simulink model "Wind_Turbine"  (R2023a)
settings: Solver=VariableStepAuto  StartTime=0.0  StopTime=20000000  FixedStep=3600  RelTol=1e-2  AbsTol=1e-2  EnableMultiTasking=on
PreLoadFcn:
  | warning off Simulink:Commands:LoadMdlParameterizedLink
PostLoadFcn:
  | warning off Simulink:blocks:MatchingGotoNotFound
  | warning off Simulink:blocks:MatchingFromNotFound
  | warning('off','Simulink:SL_OutputNotConnected');
  | warning off Simulink:Engine:SaveWithParameterizedLinks_Warning
  | warning off Simulink:Engine:SaveWithDisabledLinks_Warning
  | warning('off','Simulink:fixpoint:fxpParameterPrecisionLoss');
  | warning off Simulink:blocks:DTConversionUncessary
  | warning off ne_sli:simulator:input:FilteredInputs
  | warning off MATLAB:nearlySingularMatrix
  | 
  | warning off xPCTarget:modeloptions:StackIncrease
  | warning off xPCTarget:sampleTime:sampleTimeInvariance
  | warning off Simulink:blocks:TDelayFixedBuffer
  | 
  | Setup_WT_Configurations
StartFcn:
  | tic
StopFcn:
  | Elapsed_Sim_Time = toc;
  | disp(['Elapsed time is ' num2str(Elapsed_Sim_Time)]);
undefined symbols (not defined in the file): Actuator_Lookup, radps2rpm, sigbuilder_block, WT_Params, X, Y, Z
libraries: sm_lib x6, fl_lib x5, Wind_Lib x4, nesl_utility x4, Yaw_System_Lib x4, Pitch_System_Lib x3, Pitch_Controller_Lib x3, spsGroundLib x2, spsThreePhaseVIMeasurementLib x2, Geartrain_Lib x2, spsThreePhaseSeriesRLCLoadLib x2, spsThreePhaseBreakerLib x2
(part 2 of 2)

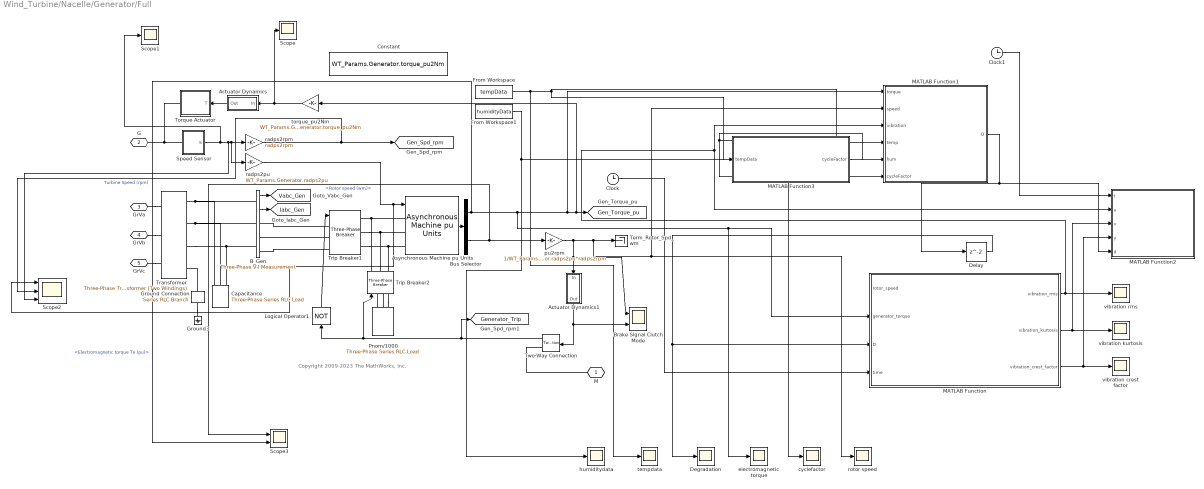
== system Wind_Turbine/Nacelle/Generator/Full ==
  note: Copyright 2009-2023 The MathWorks, Inc.
  Actuator Dynamics : Subsystem  mask(First-order lag supporting vector signals){b=WT_Params.Generator.generator_time_constant, x_initial=0}
      mask prompts: b "Filter time constant"; x_initial "Initial output"
      mask help: Models a lag of the form 1/(b*s+1) where s is the Laplace operator.
  Actuator Dynamics1 : Subsystem  mask(First-order lag supporting vector signals){b=WT_Params.Generator.generator_time_constant, x_initial=0}
      mask prompts: b "Filter time constant"; x_initial "Initial output"
      mask help: Models a lag of the form 1/(b*s+1) where s is the Laplace operator.
  Asynchronous Machine pu Units : spsAsynchronousMachinepuUnitsLib/Asynchronous Machine pu Units  RotorType=Squirrel-cage  PresetModel=No  MechanicalLoad=Speed w  ShowDetailedParameters=on  ReferenceFrame=Rotor  Units=pu  MeasurementBus=off  NominalParameters="[WT_Params.Generator.nominal_power  WT_Params.Generator.voltage WT_Params.Generator.frequency]"  VoltageRatio=1  Stator=[WT_Params.Generator.Stator.resistance WT_Params.Generator.Stator.inductance]  Rotor=[WT_Params.Generator.Rotor.resistance WT_Params.Generator.Rotor.inductance]  Cage1=[0.01909 0.0397]  Cage2=[0.01909 0.0397]  Lm=WT_Params.Generator.mutual_inductance  Mechanical=[0.09526 0.05479 3]  PolePairs=3  InitialConditions=[1 0 0 0 0 0 0 0]  SimulateSaturation=off  Saturation="[0.212,0.4201,0.8125,1.0979,1.4799,2.2457,3.2586,4.5763,6.4763 ;   0.5,0.7,0.9,1,1.1,1.2 ,1.3,1.4,1.5]"  LoadFlowParameters=1650000  TsPowergui=0  TsBlock=-1  IterativeModel=Forward Euler  IterativeDiscreteModel=Trapezoidal non iterative  Pmec=0
  B_Gen : spsThreePhaseVIMeasurementLib/Three-Phase V-I Measurement  VoltageMeasurement=phase-to-ground  SetLabelV=off  LabelV=Vabc  Vpu=on  VpuLL=off  CurrentMeasurement=yes  SetLabelI=off  LabelI=Iabc  Ipu=on  Pbase=WT_Params.Generator.nominal_power  Vbase=WT_Params.Generator.voltage  OutputType=Complex  PhasorSimulation=on  PSBequivalent=0
  Brake Signal Clutch Mode : Scope  NumInputPorts=2
  Bus Selector : BusSelector  OutputSignals=Mechanical.Electromagnetic torque Te (pu),Mechanical.Rotor speed (wm)
  Capacitance : spsThreePhaseSeriesRLCLoadLib/Three-Phase Series RLC Load  LConnTagsString=A|B|C  Configuration=Delta  NominalVoltage=WT_Params.Generator.voltage  Vabc=[1e3 1e3 1e3]  Vabcp=[1e3 1e3 1e3]  NominalFrequency=WT_Params.Generator.frequency  UnbalancedPower=off  ActivePower=0  InductivePower=0  CapacitivePower=200e3  Pabc=[10e3 9e3 11e3]  QLabc=[100 90 110]  QCabc=[100 90 110]  Pabcp=[10e3 9e3 11e3]  QLabcp=[100 90 110]  QCabcp=[100 90 110]  Measurements=None  LoadType=constant Z
  Clock : Clock
  Clock1 : Clock
  Constant : Constant  Value=WT_Params.Generator.torque_pu2Nm
  Degradation : Scope
  Delay : Delay  SampleTime=3600
  From Workspace : FromWorkspace  VariableName=tempData
  From Workspace1 : FromWorkspace  VariableName=humidityData
  Ground Connection : spsSeriesRLCBranchLib/Series RLC Branch  LConnTagsString=__new0  RConnTagsString=__new0  BranchType=R  Resistance=10  Inductance=1.0  SetiL0=off  InitialCurrent=0  Capacitance=1.0  Setx0=off  InitialVoltage=0  Measurements=None
  Ground3 : spsGroundLib/Ground  LConnTagsString=a
  Logical Operator1 : Logic  Operator=NOT  AllPortsSameDT=off  OutDataTypeStr=float('double')  SampleTime=0
  MATLAB Function : MATLAB Function  TreatAsAtomicUnit=on
  MATLAB Function1 : MATLAB Function  TreatAsAtomicUnit=on
  MATLAB Function2 : MATLAB Function  TreatAsAtomicUnit=on
  MATLAB Function3 : MATLAB Function  TreatAsAtomicUnit=on
  Pnom/1000 : spsThreePhaseSeriesRLCLoadLib/Three-Phase Series RLC Load  LConnTagsString=A|B|C  Configuration=Y (grounded)  NominalVoltage=WT_Params.Generator.voltage  Vabc=[1e3 1e3 1e3]  Vabcp=[1e3 1e3 1e3]  NominalFrequency=WT_Params.Generator.frequency  UnbalancedPower=off  ActivePower=WT_Params.Generator.nominal_power  InductivePower=0  CapacitivePower=0  Pabc=[10e3 9e3 11e3]  QLabc=[100 90 110]  QCabc=[100 90 110]  Pabcp=[10e3 9e3 11e3]  QLabcp=[100 90 110]  QCabcp=[100 90 110]  Measurements=None  LoadType=constant Z
  Scope : Scope
  Scope1 : Scope
  Scope2 : Scope  NumInputPorts=3
  Scope3 : Scope  NumInputPorts=2
  Speed Sensor : Subsystem
      mask Display:
      | plot([149.600878633536;150.016472378793;150.47508104106;150.972287968219;151.50330478576;152.063017511447;152.646035805762;153.246744883819;153.859359588817;154.477980106257;155.096648782383;155.709407499646;156.310355056631;156.893703999851;157.453836360095;157.985357756531;158.483149347555;158.942417128023;159.358738098149;159.728102859405;160.046954227227;160.312221488639;160.521349974904;160.672325664379;160.763694578642;160.794576785101;160.764674871227;160.674276808796;160.524253180566;160.316048796087;160.051668777399;159.733659248606;159.365082815313;158.949489070056;158.490880407788;157.993673480629;157.462656663088;156.908284800231], [156.971389291536;157.430657072004;157.84697804213;158.216342803387;158.535194171208;158.80046143262;159.009589918885;159.16056560836;159.251934522623;159.282816729083;159.252914815208;159.162516752777;159.012493124547;158.804288740068;158.53990872138;158.221899192587;157.853322759294;157.437729014037;156.979120351769;156.48191342461;155.950896607069;155.391183881382;154.808165587067;154.20745650901;153.594841804012;152.976221286573;152.357552610446;151.744793893183;151.143846336199;150.560497392978;150.000365032735;149.468843636298;148.971052045274;148.511784264806;148.095463294681;147.726098533424;147.407247165603;147.144199990631])
      | plot([152.057635404444;152.93604260309;153.834625296826;154.744729643097;155.657590839533;156.564417533794;157.45647648909;158.325176690034;159.162152078811;159.959342124889;160.709069452336;161.404113777147;162.037781442523;162.603969882449;163.097226392739;163.512800643557;163.846690427691;164.095680203997;164.257372064819;164.330208829146;164.313489039122;164.27939575172], [142.228020686971;141.979030910664;141.817339049842;141.744502285515;141.761222075539;141.867337399197;142.061826307913;142.342815767178;142.707599694895;143.152665022428;143.673725527376;144.265763112236;144.923076131425;145.639334301243;146.40763966397;147.220593018964;148.070365181011;148.948772379657;149.847355073393;150.757459419663;151.6703206161;152.055850472277])
      | plot([116.468514315784;116.438789536125;116.349901463023;116.202706137216;115.998621130155;115.739611892022;115.42817282337;115.067303252679;114.660478551187;114.211616663162;113.725040373958;113.205435679231;112.657806656235;112.087427271827;111.499790591278;110.900555877058;110.29549408704;109.690432297022;109.091197582803;108.503560902254;107.933181517846;107.38555249485;106.865947800123;106.379371510919;105.930509622894;105.523684921402;105.162815350711;104.851376282059;104.592367043926;104.388282036865;104.241086711057;104.152198637956;104.122473858297;104.152198637956;104.241086711057;104.388282036865;104.592367043926;104.851376282059;105.162815350711;105.523684921402;105.930509622894;106.379371510919;106.865947800123;107.38555249485;107.933181517846;108.503560902254;109.091197582803;109.690432297022;110.29549408704;110.900555877058;111.499790591278;112.087427271827;112.657806656235;113.205435679231;113.725040373958;114.211616663162;114.660478551187;115.067303252679;115.42817282337;115.739611892022;115.998621130155;116.202706137216;116.349901463023;116.438789536125;116.468514315784;116.468514315784], [111.618284136057;111.013222346039;110.413987631819;109.826350951271;109.255971566862;108.708342543866;108.188737849139;107.702161559936;107.253299671911;106.846474970419;106.485605399728;106.174166331075;105.915157092943;105.711072085881;105.563876760074;105.474988686973;105.445263907313;105.474988686973;105.563876760074;105.711072085881;105.915157092943;106.174166331075;106.485605399728;106.846474970419;107.253299671911;107.702161559936;108.188737849139;108.708342543866;109.255971566862;109.826350951271;110.413987631819;111.013222346039;111.618284136057;112.223345926075;112.822580640295;113.410217320843;113.980596705252;114.528225728247;115.047830422975;115.534406712178;115.983268600203;116.390093301695;116.750962872386;117.062401941038;117.321411179171;117.525496186232;117.67269151204;117.761579585141;117.7913043648;117.761579585141;117.67269151204;117.525496186232;117.321411179171;117.062401941038;116.750962872386;116.390093301695;115.983268600203;115.534406712178;115.047830422975;114.528225728247;113.980596705252;113.410217320843;112.822580640295;112.223345926075;111.618284136057;111.618284136057])
      | plot([239.23602886498;238.828071429858;237.608127977604;235.587947230552;232.78698463364;229.232214987837;224.957872668068;220.005121927465;214.421660463109;208.261260061133;201.583248745024;194.451939414329;186.936010476274;179.107844435155;171.042830809261;162.818640088593;154.514475725591;146.210311362589;137.986120641921;129.921107016027;122.092940974909;114.577012036853;107.445702706158;100.76769139005;94.607290988073;89.0238295237172;84.0710787831142;79.7967364633452;76.2419668175427;73.4410042206305;71.4208234735788;70.2008800213248;69.7929225862026;70.2008800213248;71.4208234735788;73.4410042206306;76.2419668175428;79.7967364633454;84.0710787831144;89.0238295237174;94.6072909880733;100.76769139005;107.445702706159;114.577012036853;122.092940974909;129.921107016027;137.986120641921;146.210311362589;154.514475725591;162.818640088593;171.042830809261;179.107844435155;186.936010476274;194.451939414329;201.583248745024;208.261260061133;214.421660463109;220.005121927465;224.957872668068;229.232214987837;232.78698463364;235.587947230552;237.608127977604;238.828071429858;239.23602886498;239.23602886498], [155.774275772274;147.47628550917;139.258209428443;131.199192095207;123.376846251889;115.866505365088;108.740498123116;102.067451871182;95.9116316925529;90.3323215006612;85.3832531026163;81.1120887325275;77.5599620381344;74.7610819412943;72.742403187363;71.5233667562631;71.1157126352191;71.5233667562631;72.742403187363;74.7610819412943;77.5599620381345;81.1120887325275;85.3832531026164;90.3323215006612;95.9116316925529;102.067451871182;108.740498123116;115.866505365089;123.376846251889;131.199192095207;139.258209428443;147.47628550917;155.774275772274;164.072266035377;172.290342116104;180.34935944934;188.171705292658;195.682046179459;202.808053421432;209.481099673365;215.636919851994;221.216230043886;226.165298441931;230.43646281202;233.988589506413;236.787469603253;238.806148357184;240.025184788284;240.432838909328;240.025184788284;238.806148357184;236.787469603253;233.988589506413;230.43646281202;226.165298441931;221.216230043886;215.636919851994;209.481099673365;202.808053421432;195.682046179459;188.171705292658;180.34935944934;172.290342116105;164.072266035378;155.774275772274;155.774275772274])
      | plot([252.715889364481;252.243022716633;250.828976737403;248.487369462568;245.240751850236;241.120390602797;236.165967051481;230.425195003451;223.953361231755;216.812793033479;209.072257983804;200.806301666664;192.094529760025;183.020841389688;173.672621134841;164.139897466795;154.514475725591;144.889053984387;135.356330316341;126.008110061494;116.934421691157;108.222649784518;99.9566934673787;92.2161584177032;85.075590219427;78.6037564477313;72.8629843997015;67.9085608483856;63.7881996009461;60.5415819886144;58.199974713779;56.7859287345493;56.3130620867014;56.7859287345493;58.1999747137791;60.5415819886146;63.7881996009463;67.9085608483858;72.8629843997018;78.6037564477315;85.0755902194273;92.2161584177035;99.9566934673791;108.222649784519;116.934421691157;126.008110061494;135.356330316341;144.889053984387;154.514475725591;164.139897466796;173.672621134841;183.020841389688;192.094529760025;200.806301666664;209.072257983803;216.812793033479;223.953361231755;230.425195003451;236.165967051481;241.120390602797;245.240751850236;248.487369462568;250.828976737403;252.243022716633;252.715889364481;252.715889364481], [154.514475725591;144.895228084285;135.36861905618;126.026395093992;116.958526921455;108.252343066071;99.9916888376535;92.2561188521535;85.1201308772245;78.6524483779929;72.9153586725213;67.9641130708855;63.8463947748555;60.6018596625959;58.2617543808809;56.8486154228053;56.3760520890355;56.8486154228053;58.2617543808809;60.6018596625959;63.8463947748555;67.9641130708856;72.9153586725213;78.652448377993;85.1201308772246;92.2561188521536;99.9916888376536;108.252343066072;116.958526921455;126.026395093992;135.36861905618;144.895228084285;154.514475725591;164.133723366898;173.660332395002;183.002556357191;192.070424529728;200.776608385111;209.037262613529;216.772832599029;223.908820573958;230.37650307319;236.113592778661;241.064838380297;245.182556676327;248.427091788587;250.767197070302;252.180336028377;252.652899362147;252.180336028377;250.767197070301;248.427091788587;245.182556676327;241.064838380297;236.113592778661;230.37650307319;223.908820573958;216.772832599029;209.037262613529;200.776608385111;192.070424529728;183.002556357191;173.660332395002;164.133723366898;154.514475725592;154.514475725591])
      | plot([154.514475725591;129.948374815285;179.017586633563;154.514475725591], [240.369848906994;203.583687543869;203.583687543869;240.369848906994])
      | plot([105.382273904979;149.60125554353], [115.271704271436;156.971085816622])
      | plot([144.688035361469;144.688035361469], [152.057865634561;203.583687543869])
      | plot([164.277926087379;164.277926087379], [152.057865634561;203.583687543869])
      | plot([159.112745895982;159.616665914655], [149.60125554353;149.60125554353])
      | plot([115.208714269102;159.364705905318], [107.901873998344;149.60125554353])
      | plot([0;311.800511553884;311.800511553884;0;0], [311.800511553884;311.800511553884;0;0;311.800511553884])
      | ;
      | color('red');
      | port_label('LConn', 1,'R')
      | port_label('output', 1,'W')
  Term_Rotor_Spd_wm : Terminator
  Torque Actuator : Subsystem
      mask Display:
      | plot([198.657636314574;187.5372000791;176.524559560751;165.725772507838;155.244837142898;145.182690602959;135.636236859729;126.697413481378;118.452306223496;110.980319976212;104.353414051689;98.6354091766174;93.8813728637222;90.1370890815176;87.4386173296598;85.811945366254;85.272738931537;85.8261908782356;87.4669711615554;90.1792781704262;93.9369909056548;98.7039205394262;104.434158933498;111.072520759669;118.555074964656;126.809760461083;135.75708011515;145.310866347487;155.379110974044;165.864851295207;176.667103899592;187.681837189509;192.988368326926], [283.691199740558;283.13774779386;281.49696751054;278.784660501669;275.026947766441;270.260018132669;264.529779738597;257.891417912426;250.40886370744;242.154178211013;233.206858556945;223.653072324609;213.584827698051;203.099087376889;192.296834772503;181.282101482586;170.160965409986;159.040529174513;148.027888656163;137.22910160325;126.748166238311;116.686019698372;107.139565955142;98.2007425767901;89.9556353189084;82.4836490716241;75.8567431471018;70.1387382720299;65.3847019591348;61.6404181769301;58.9419464250722;57.3152744616664;56.9214337615639])
      | plot([85.209725657478;1.11807254143059;1.11807254143059], [170.435198815539;170.435198815539;171.380048850551])
      | plot([283.691223012283;397.073227213696], [170.309218810871;170.309218810871])
      | plot([153.301918180659;255.34572196193], [170.309218810871;170.309218810871])
      | plot([198.654719861224;113.618216710165;198.654719861224], [85.2727156598121;170.309218810871;255.34572196193])
      | plot([198.654719861224;153.301918180659;198.654719861224], [215.662020491436;170.309218810871;124.956417130306])
      | plot([198.654719861224;283.691223012283;283.691223012283;187.316519441083;192.985619651154], [283.691223012283;283.691223012283;56.927214609459;56.927214609459;56.927214609459])
      | 
      | patch([395.419739652425;395.419739652425;5.6843418860808e-14;0;395.419739652425;394.947314634919;0.472425017505884;0.472425017505941;394.947314634919;394.947314634919;395.419739652425], [340.618437621742;5.6843418860808e-14;0;340.618437621742;340.618437621742;340.146012604237;340.146012604237;0.472425017505884;0.472425017505884;340.146012604237;340.618437621742], [1;1;1])
      | ;
      | color('red');
      | port_label('RConn', 1,'R')
      | port_label('Input', 1,'T')
  Transformer : spsThreePhaseTransformerTwoWindingsLib/Three-Phase Transformer (Two Windings)  Winding1Connection=Yg  Winding2Connection=Yn  CoreType=Three single-phase transformers  SetSaturation=off  Hysteresis=off  DataFile='hysteresis'  SetInitialFlux=off  Measurements=None  UNITS=pu  NominalPower="[2e6  60]"  Winding1=[WT_Params.Grid.voltage, 0.025/30 , 0.025]  Winding2=[ WT_Params.Generator.voltage, 0.025/30 , 0.025]  Rm=500  Lm=inf  L0=0.5  Saturation=[ 0,0 ; 0.0024,1.2 ; 1.0,1.52 ]  InitialFluxes=[ 0.8 , -0.8 , 0.7 ]  BreakLoop=off  DiscreteSolver=Trapezoidal iterative  DataType=off  TransfoNumber=0
  Trip Breaker1 : spsThreePhaseBreakerLib/Three-Phase Breaker  InitialState=closed  SwitchA=on  SwitchB=on  SwitchC=on  SwitchTimes="[4/60  10/60]"  External=on  BreakerResistance=WT_Params.Generator.Breakers.ron  SnubberResistance=WT_Params.Generator.Breakers.rp  SnubberCapacitance=WT_Params.Generator.Breakers.cp  Measurements=None
  Trip Breaker2 : spsThreePhaseBreakerLib/Three-Phase Breaker  InitialState=open  SwitchA=on  SwitchB=on  SwitchC=on  SwitchTimes="[4/60  10/60]"  External=on  BreakerResistance=WT_Params.Generator.Breakers.ron  SnubberResistance=WT_Params.Generator.Breakers.rp  SnubberCapacitance=WT_Params.Generator.Breakers.cp  Measurements=None
  Two-Way Connection : TwoWayConnection
  cyclefactor : Scope
  electromagnetic torque : Scope
  humiditydata : Scope
  pu2rpm : Gain  Gain=1/WT_Params.Generator.radps2pu*radps2rpm
  radps2pu : Gain  Gain=WT_Params.Generator.radps2pu
  radps2rpm : Gain  Gain=radps2rpm
  rotor speed : Scope
  tempdata : Scope
  torque_pu2Nm : Gain  Gain=WT_Params.Generator.torque_pu2Nm
  vibration crest factor : Scope
  vibration kurtosis : Scope
  vibration rms : Scope
  M : PMIOPort  Tag=PMCPort  Side=Left
  G : PMIOPort  Port=2  Side=Left
  GrVa : PMIOPort  Port=3  Side=Right
  GrVb : PMIOPort  Port=4  Side=Right
  GrVc : PMIOPort  Port=5  Side=Right
  tag scope: Gen_Spd_rpm=global, Gen_Torque_pu=global, Generator_Trip=global, Iabc_Gen=global, Vabc_Gen=global
  wires:
  Actuator Dynamics1/1(Out) -> Two-Way Connection/1, Brake Signal Clutch Mode/2
  Actuator Dynamics/1(Out) -> Torque Actuator/1(T)
  B_Gen/2 -> [Iabc_Gen]
  B_Gen/1 -> [Vabc_Gen]
  Asynchronous Machine pu Units/1 -> Bus Selector/1
  Speed Sensor/1(S) -> Scope1/1, Scope2/3, radps2rpm/1, radps2pu/1
  Bus Selector/1 -> Scope3/2, MATLAB Function1/1(torque), torque_pu2Nm/1, [Gen_Torque_pu], electromagnetic torque/1, MATLAB Function/2(generator_torque)  "<Electromagnetic torque Te (pu)>"
  radps2pu/1 -> Scope2/1, Asynchronous Machine pu Units/1
  torque_pu2Nm/1 -> Scope/1, Actuator Dynamics/1(In)
  radps2rpm/1 -> Scope2/2, [Gen_Spd_rpm]  "Turbine Speed (rpm)"
  Bus Selector/2 -> Scope3/1, pu2rpm/1  "<Rotor speed (wm)>"
  pu2rpm/1 -> MATLAB Function1/2(speed), rotor speed/1, Term_Rotor_Spd_wm/1, Actuator Dynamics1/1(In), Brake Signal Clutch Mode/1
  Two-Way Connection/1 -> [Generator_Trip], Trip Breaker2/1, Logical Operator1/1
  Logical Operator1/1 -> Trip Breaker1/1
  Delay/1 -> MATLAB Function/3(D), Degradation/1
  Clock/1 -> MATLAB Function/4(time)
  MATLAB Function/1(vibration_rms) -> vibration rms/1, MATLAB Function2/2(u), MATLAB Function1/3(vibration)
  From Workspace/1 -> tempdata/1, MATLAB Function1/4(temp), MATLAB Function3/1(tempData)
  From Workspace1/1 -> humiditydata/1, MATLAB Function1/5(hum)
  MATLAB Function1/1(D) -> Delay/1, MATLAB Function2/5(d)
  Clock1/1 -> MATLAB Function2/1(t)
  MATLAB Function/2(vibration_kurtosis) -> vibration kurtosis/1, MATLAB Function2/3(v)
  MATLAB Function/3(vibration_crest_factor) -> vibration crest factor/1, MATLAB Function2/4(y)
  MATLAB Function3/1(cycleFactor) -> cyclefactor/1, MATLAB Function1/6(cycleFactor)
  connections:
  Transformer/RConn2 -- B_Gen/LConn2 -- Capacitance/LConn2
  M/RConn1 -- Two-Way Connection/RConn1
  Transformer/RConn1 -- B_Gen/LConn1 -- Capacitance/LConn1
  Transformer/RConn3 -- B_Gen/LConn3 -- Capacitance/LConn3
  Speed Sensor/LConn1 -- G/RConn1 -- Torque Actuator/RConn1
  GrVb/RConn1 -- Transformer/LConn2
  GrVc/RConn1 -- Transformer/LConn3
  GrVa/RConn1 -- Transformer/LConn1
  Ground Connection/RConn1 -- Ground3/LConn1
  Ground Connection/LConn1 -- Transformer/RConn4
  Pnom/1000/LConn1 -- Trip Breaker2/LConn1
  Trip Breaker2/LConn3 -- Pnom/1000/LConn3
  Pnom/1000/LConn2 -- Trip Breaker2/LConn2
  Trip Breaker1/RConn3 -- Asynchronous Machine pu Units/LConn3 -- Trip Breaker2/RConn3
  Trip Breaker1/RConn2 -- Asynchronous Machine pu Units/LConn2 -- Trip Breaker2/RConn2
  Asynchronous Machine pu Units/LConn1 -- Trip Breaker1/RConn1 -- Trip Breaker2/RConn1
  Trip Breaker1/LConn3 -- B_Gen/RConn3
  Trip Breaker1/LConn2 -- B_Gen/RConn2
  Trip Breaker1/LConn1 -- B_Gen/RConn1

== system Wind_Turbine/Scopes/Configure Turbine/Subsystem ==

== system Wind_Turbine/Scopes/Configure Turbine/Subsystem1 ==

== system Wind_Turbine/Scopes/Configure Turbine/Subsystem10 ==

== system Wind_Turbine/Scopes/Configure Turbine/Subsystem11 ==

== system Wind_Turbine/Scopes/Configure Turbine/Subsystem12 ==

== system Wind_Turbine/Scopes/Configure Turbine/Subsystem13 ==

== system Wind_Turbine/Scopes/Configure Turbine/Subsystem14 ==

== system Wind_Turbine/Scopes/Configure Turbine/Subsystem15 ==

== system Wind_Turbine/Scopes/Configure Turbine/Subsystem16 ==

== system Wind_Turbine/Scopes/Configure Turbine/Subsystem17 ==

== system Wind_Turbine/Scopes/Configure Turbine/Subsystem18 ==

== system Wind_Turbine/Scopes/Configure Turbine/Subsystem19 ==

== system Wind_Turbine/Scopes/Configure Turbine/Subsystem2 ==

== system Wind_Turbine/Scopes/Configure Turbine/Subsystem20 ==

== system Wind_Turbine/Scopes/Configure Turbine/Subsystem21 ==

== system Wind_Turbine/Scopes/Configure Turbine/Subsystem22 ==

== system Wind_Turbine/Scopes/Configure Turbine/Subsystem23 ==

== system Wind_Turbine/Scopes/Configure Turbine/Subsystem24 ==

== system Wind_Turbine/Scopes/Configure Turbine/Subsystem3 ==

== system Wind_Turbine/Scopes/Configure Turbine/Subsystem4 ==

== system Wind_Turbine/Scopes/Configure Turbine/Subsystem5 ==

== system Wind_Turbine/Scopes/Configure Turbine/Subsystem6 ==

== system Wind_Turbine/Scopes/Configure Turbine/Subsystem7 ==

== system Wind_Turbine/Scopes/Configure Turbine/Subsystem8 ==

== system Wind_Turbine/Scopes/Configure Turbine/Subsystem9 ==

== system Wind_Turbine/Turbine Input/Commands/Signal Builder ==
  Demux : Demux  Tag=STV Demux  Outputs=1
      settings: DisplayOption=none
  FromWs : FromWorkspace  Tag=STV FromWs  VariableName=tuvar
      SigBuilderData=|
      | common.afterFinalStr = 'Extrapolate'
      | common.sampleTime = 0
      | dataSet(1).timeRange = [0 50]
      | dataSet(1).name = 'Pos_Test'
      | dataSet(2).timeRange = [0 50]
      | dataSet(2).name = 'Pos_Neg_Test'
      | dataSet(3).timeRange = [0 50]
      | dataSet(3).name = 'Step_Test'
      | sbobj.Groups(1).Name = 'Pos_Test'
      | sbobj.Groups(1).Signals.Name = 'Signal 1'
      | sbobj.Groups(1).Signals.XData = [0 5 5 7.5 7.5 25.1 25.1 28 28 50]
      | sbobj.Groups(1).Signals.YData = [0 0 20 20 0 0 20 20 0 0]
      | sbobj.Groups(1).TimeRange = [0 50]
      | sbobj.Groups(2).Name = 'Pos_Neg_Test'
      | sbobj.Groups(2).Signals.Name = 'Signal 1'
      | sbobj.Groups(2).Signals.XData = [0 3 3 5.5 5.5 8 8 10.5 10.5 50]
      | sbobj.Groups(2).Signals.YData = [0 0 20 20 0 0 -20 -20 0 0]
      | sbobj.Groups(2).TimeRange = [0 50]
      | sbobj.Groups(3).Name = 'Step_Test'
      | sbobj.Groups(3).Signals.Name = 'Signal 1'
      | sbobj.Groups(3).Signals.XData = [0 1 1 7.5 25.1 30 30 50]
      | sbobj.Groups(3).Signals.YData = [0 0 20 20 20 20 0 0]
      | sbobj.Groups(3).TimeRange = [0 50]
  Signal 1 : Outport  Tag=STV Outport  VectorParamsAs1DForOutWhenUnconnected=off
  wires:
  Demux/1 -> Signal 1/1
  FromWs/1 -> Demux/1

== system Wind_Turbine/Turbine Input/Commands/Signal Builder2 ==
  Demux : Demux  Tag=STV Demux  Outputs=1
      settings: DisplayOption=none
  FromWs : FromWorkspace  Tag=STV FromWs  VariableName=tuvar
      SigBuilderData=|
      | common.afterFinalStr = 'Extrapolate'
      | common.sampleTime = 0
      | dataSet(1).timeRange = [0 50]
      | dataSet(1).name = 'Pos_Neg_Test'
      | dataSet(2).timeRange = [0 50]
      | dataSet(2).name = 'Step_Test'
      | dataSet(3).timeRange = [0 50]
      | dataSet(3).name = 'Ramp_Test'
      | sbobj.Groups(1).Name = 'Pos_Neg_Test'
      | sbobj.Groups(1).Signals.Name = 'Signal 1'
      | sbobj.Groups(1).Signals.XData = [0 1 1 11 11 21 21 31 31 50]
      | sbobj.Groups(1).Signals.YData = [0 0 4 4 0 0 -4 -4 0 0]
      | sbobj.Groups(2).Name = 'Step_Test'
      | sbobj.Groups(2).Signals.Name = 'Signal 1'
      | sbobj.Groups(2).Signals.XData = [0 1 1 11 21 31 31 50]
      | sbobj.Groups(2).Signals.YData = [0 0 4 4 4 4 0 0]
      | sbobj.Groups(3).Name = 'Ramp_Test'
      | sbobj.Groups(3).Signals.Name = 'Signal 1'
      | sbobj.Groups(3).Signals.XData = [0 1 1 11 21 31 39.1 50]
      | sbobj.Groups(3).Signals.YData = [0 0 2.46 4 2.32 3.18 1.16 0]
  Signal 1 : Outport  Tag=STV Outport  VectorParamsAs1DForOutWhenUnconnected=off
  wires:
  Demux/1 -> Signal 1/1
  FromWs/1 -> Demux/1

== system Wind_Turbine/Nacelle/Generator/Full/Actuator Dynamics ==
  In : Inport
  Gain : Gain  Gain=1/b
  Integrator : Integrator  InitialCondition=x_initial
  Sum : Sum  Inputs=|+-  InputSameDT=on  SaturateOnIntegerOverflow=on  OutDataTypeStr=Inherit: Same as first input
  Out : Outport  VectorParamsAs1DForOutWhenUnconnected=off
  wires:
  Sum/1 -> Integrator/1
  In/1 -> Sum/1
  Integrator/1 -> Gain/1
  Gain/1 -> Sum/2, Out/1

== system Wind_Turbine/Nacelle/Generator/Full/Actuator Dynamics1 ==
  In : Inport
  Gain : Gain  Gain=1/b
  Integrator : Integrator  InitialCondition=x_initial
  Sum : Sum  Inputs=|+-  InputSameDT=on  SaturateOnIntegerOverflow=on  OutDataTypeStr=Inherit: Same as first input
  Out : Outport  VectorParamsAs1DForOutWhenUnconnected=off
  wires:
  Gain/1 -> Out/1, Sum/2
  Integrator/1 -> Gain/1
  In/1 -> Sum/1
  Sum/1 -> Integrator/1

== system Wind_Turbine/Nacelle/Generator/Full/Speed Sensor ==
  Ideal Rotational Motion Sensor : fl_lib/Mechanical/Mechanical Sensors/Ideal Rotational Motion Sensor  reference=foundation.enum.MeasurementReference.difference  acceleration_port=false  velocity_port=true  position_port=true  wrap_angle=simscape.enum.onoff.off  offset=0 rad
  Mechanical Rotational Reference1 : fl_lib/Mechanical/Rotational Elements/Mechanical Rotational Reference
  PS-Simulink Converter : nesl_utility/PS-Simulink Converter  PhysicalDomain=network_engine_domain  SubClassName=ps_output  LeftPortType=input  RightPortType=output  PseudoPeriodic=off  Frequencies=[]  VectorFormat=1-D array  Unit=rad/s  AffineConversion=off
  R : PMIOPort  Side=Left
  S : Outport  VectorParamsAs1DForOutWhenUnconnected=off
  wires:
  PS-Simulink Converter/1 -> S/1
  connections:
  Mechanical Rotational Reference1/LConn1 -- Ideal Rotational Motion Sensor/RConn1
  R/RConn1 -- Ideal Rotational Motion Sensor/LConn1
  Ideal Rotational Motion Sensor/RConn2 -- PS-Simulink Converter/LConn1

== system Wind_Turbine/Nacelle/Generator/Full/Torque Actuator ==
  T : Inport
  Ideal Torque Source : fl_lib/Mechanical/Mechanical Sources/Ideal Torque Source
  Mechanical Rotational Reference : fl_lib/Mechanical/Rotational Elements/Mechanical Rotational Reference
  Simulink-PS Converter : nesl_utility/Simulink-PS Converter  PhysicalDomain=network_engine_domain  SubClassName=ps_input  LeftPortType=input  RightPortType=output  PseudoPeriodic=off  Frequencies=[]  NoiseDistribution=none  NoiseParameters=[]  Unit=1  AffineConversion=off  FilteringAndDerivatives=filter  SimscapeFilterOrder=1  InputFilterTimeConstant=0.005  UdotUserProvided=1
  R : PMIOPort  Side=Right
  wires:
  T/1 -> Simulink-PS Converter/1
  connections:
  R/RConn1 -- Ideal Torque Source/LConn1
  Mechanical Rotational Reference/LConn1 -- Ideal Torque Source/RConn2
  Simulink-PS Converter/RConn1 -- Ideal Torque Source/RConn1

== matlab function Wind_Turbine/Nacelle/Generator/Full/MATLAB Function ==
  settings: updateMethod=DISCRETE  sampleTime=3600
  data: rotor_speed input; vibration_rms output; generator_torque input; D input; time input; vibration_kurtosis output; vibration_crest_factor output
function [vibration_rms, vibration_kurtosis, vibration_crest_factor] = generator_vibration_sensor(rotor_speed, generator_torque, D, time)
% Updated function with better kurtosis handling over a moving window

% Convert degradation to health
generator_health = max(0.01, min(1, 1 - D));

% Parameters
torque_sensitivity = 0.05;
speed_sensitivity = 0.03;
noise_amplitude = 0.1;
wear_factor = 1 + (1 - generator_health) * 3;
fault_time = 300;
fault_magnitude = 0.5;

% Compute base signal
base_vibration = torque_sensitivity * generator_torque + speed_sensitivity * rotor_speed;
noise = noise_amplitude * wear_factor * randn();
fault = (time > fault_time) * fault_magnitude * (1 - generator_health) * sin(2*pi*5*time);

% Final vibration sample
vibration_sample = base_vibration + noise + fault;

% --- Persistent buffer for windowed analysis ---
persistent buffer
buffer_size = 100;  % e.g., 100 samples for kurtosis
if isempty(buffer)
    buffer = zeros(1, buffer_size);
end

% Shift buffer and add new sample
buffer = [buffer(2:end), vibration_sample];

% Compute features
vibration_rms = sqrt(mean(vibration_sample.^2));  % Still single sample RMS
vibration_kurtosis = kurtosis(buffer);  % Now over buffer
vibration_crest_factor = max(abs(buffer)) / (vibration_rms + eps);

end

== matlab function Wind_Turbine/Turbine Input/Wind/MATLAB Function ==
  data: t input; ws output; speedVec input; dirVec input; wd output
function [ws, wd] = fcn(t, speedVec, dirVec)
%#codegen

% Assume timeVec is simply a linear time vector (e.g., 0, 1, 2, ..., N-1)
N = length(speedVec);
timeVec = (0:N-1)';

% Make sure vectors are column vectors
speedVec = speedVec(:);
dirVec = dirVec(:);

% Find the index of the closest time point
[~, idx] = min(abs(timeVec - t));

% Lookup values safely
ws = speedVec(idx);
wd = dirVec(idx);

== matlab function Wind_Turbine/Nacelle/Generator/Full/MATLAB Function1 ==
  settings: updateMethod=DISCRETE  sampleTime=3600
  data: torque input; D output; speed input; vibration input; temp input; hum input; cycleFactor input
function D = windTurbineGeneratorDegradation(torque, speed, vibration, temp, hum, cycleFactor)
%#codegen
persistent Dval
if isempty(Dval)
    Dval = 0;
end

% Parameters 
alpha1 = 1e-8;  % mechanical base wear
alpha2 = 2e-6;  % vibration
alpha3 = 1e-7;  % temperature aging
alpha4 = 5e-8;  % humidity effect
alpha5 = 3e-7;  % thermal cycling

% Arrhenius parameters for electrical insulation
Ea = 0.8;            % Activation energy (eV) - typical for insulation
kb = 8.617e-5;       % Boltzmann constant (eV/K)
T_ref = 298.15;      % Reference temperature (25°C in Kelvin)
T_K = temp + 273.15; % Convert °C to Kelvin

% Compute Arrhenius temperature acceleration factor
tempAccFactor = exp((Ea/kb) * (1/T_ref - 1/T_K));

% Wind turbine specific components
mechWear = (abs(torque) * abs(speed))^1.2; % Non-linear relationship
vibStress = vibration^2;
thermalStress = tempAccFactor;
humidityStress = exp(0.05 * hum); % Exponential effect of humidity
cycleStress = alpha5 * cycleFactor; % Use pre-calculated cycle factor

% Total degradation step
dD = alpha1*mechWear + alpha2*vibStress + alpha3*thermalStress + alpha4*humidityStress + cycleStress;

% Update degradation (clamped to 0-1)
Dval = min(Dval + dD, 1);
D = Dval;
end

== matlab function Wind_Turbine/Nacelle/Generator/Full/MATLAB Function2 ==
  settings: updateMethod=DISCRETE  sampleTime=3600
  data: t input; u input; v input; y input; d input
function logToCSV(t, u, v, y,d)
%#codegen
persistent fid isHeaderWritten

if isempty(fid)
    fid = fopen('signal_data1.csv', 'w');  % Open file for writing
    isHeaderWritten = false;
end

% Write header once
if ~isHeaderWritten
    fprintf(fid, 'Time (s),U,V,Y\n');
    isHeaderWritten = true;
end

% Write one row of data
fprintf(fid, '%.4f,%.4f,%.4f,%.4f,%.4f\n', t, u, v, y,d);

== matlab function Wind_Turbine/Nacelle/Generator/Full/MATLAB Function3 ==
  data: tempData input; cycleFactor output
function cycleFactor = simpleCycleFactor(tempData)
%#codegen
% Simple cycle factor calculation without rainflow counting
% Works with a 1D temperature array

% Parameters
tempRangeThreshold = 5;  % Minimum temp change to count as cycle (°C)
tempRangePower = 1.5;    % Power factor for temp range
baseCycleDamage = 0.01;  % Base damage per cycle

% Find peaks and valleys (simplified cycle identification)
isPeak = zeros(size(tempData));
isValley = zeros(size(tempData));

for i = 2:length(tempData)-1
    if tempData(i) > tempData(i-1) && tempData(i) > tempData(i+1)
        isPeak(i) = 1;
    elseif tempData(i) < tempData(i-1) && tempData(i) < tempData(i+1)
        isValley(i) = 1;
    end
end

peakIndices = find(isPeak);
valleyIndices = find(isValley);


% Count cycles and their ranges
cycleCount = 0;
totalWeightedRange = 0;

% Simplified approach - just pair adjacent peaks and valleys
tempRanges = [];
for i = 1:min(length(peakIndices), length(valleyIndices))-1
    range = abs(tempData(peakIndices(i)) - tempData(valleyIndices(i)));
    if range >= tempRangeThreshold
        tempRanges(end+1) = range;
    end
end

% Weight the ranges
weightedRanges = tempRanges.^tempRangePower;
cycleFactor = sum(weightedRanges) * baseCycleDamage;

end

== stateflow chart Wind_Turbine/Main Controller/Wind Input/Turbine State Machine ==
  state Generating
    entry: parking_brake = 0;
    generator_trip = 0;
    pitch_brake = 0;
    turbine_state = 2;
  state Startup
    entry: parking_brake = 0;
    generator_trip = 1;
    pitch_brake = 0;
    turbine_state = 1;
  state Park
    entry: parking_brake = 1;
    generator_trip = 1;
    pitch_brake = 1;
    turbine_state = 0;
  state Brake
    entry: parking_brake = 0;
    generator_trip = 1;
    pitch_brake = 1;
    turbine_state = 3;
  Startup -> Generating [order 1] : [turbine_speed>...
      | turbine_speed_cut_in]
  Park -> Startup : [wind_speed>...
      | 1.1...
      | &&wind_speed<...
      | wind_speed_cut_out]
  Startup -> Brake [order 2] : [wind_speed<...
      | 1.1]
  Brake -> Startup [order 2] : [wind_speed<...
      | wind_speed_cut_in_upper...
      | && wind_speed>...
      | 1.1]
  Generating -> Brake : [wind_speed<...
      | 1.1...
      | ||wind_speed>...
      | wind_speed_cut_out...
      | ||turbine_speed>...
      | turbine_speed_cut_out...
      | ||turbine_speed<...
      | turbine_speed_cut_in*0.9]
  (default) -> Park
  Brake -> Park [order 1] : [turbine_speed<=...
      | park_speed]
  data: pitch_brake output double; wind_speed input; turbine_speed input; parking_brake output double; generator_trip output double; wind_speed_cut_in_lower local double =WT_Params.Main_Controller.wind_speed_cut_in_lower; turbine_speed_cut_in local double =WT_Params.Main_Controller.turbine_speed_cut_in; turbine_state output double; wind_speed_cut_out local double =WT_Params.Main_Controller.wind_speed_cut_out; wind_speed_cut_in_upper local double =WT_Params.Main_Controller.wind_speed_cut_in_upper; turbine_speed_cut_out local double =WT_Params.Main_Controller.turbine_speed_cut_out; park_speed constant double =WT_Params.Main_Controller.turbine_speed_park
